simulink model "M_iHGU"  (R2019a)
settings: Solver=VariableStepAuto  StartTime=0.0  StopTime=10.0  RelTol=1e-3
undefined symbols (not defined in the file): ILC_B, M_iinfHGU_aD, M_iinfHGU_bD, M_iinfHGU_cD, M_iinfHGU_dD
settings Model: Creator=rache  LastModifiedBy=rache
settings DataIOCC: ReturnWorkspaceOutputs=off
settings DebuggingCC: ArithmeticOperatorsInVariantConditions=warning

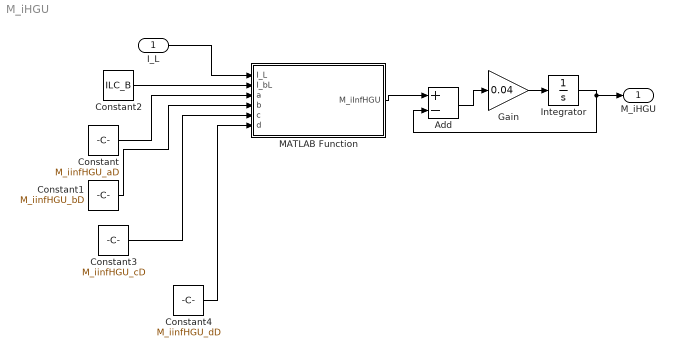
== system M_iHGU ==
  I_L : Inport
  Add : Sum  Inputs=+-
  Constant : Constant  Value=M_iinfHGU_aD
  Constant1 : Constant  Value=M_iinfHGU_bD
  Constant2 : Constant  Value=ILC_B
  Constant3 : Constant  Value=M_iinfHGU_cD
  Constant4 : Constant  Value=M_iinfHGU_dD
  Gain : Gain  Gain=0.04
  Integrator : Integrator
  MATLAB Function : MATLAB Function  TreatAsAtomicUnit=on
  M_iHGU : Outport
  wires:
  Integrator/1 -> Add/2, M_iHGU/1
  MATLAB Function/1(M_iInfHGU) -> Add/1
  Add/1 -> Gain/1
  Gain/1 -> Integrator/1
  Constant2/1 -> MATLAB Function/2(I_bL)
  I_L/1 -> MATLAB Function/1(I_L)
  Constant/1 -> MATLAB Function/3(a)
  Constant1/1 -> MATLAB Function/4(b)
  Constant3/1 -> MATLAB Function/5(c)
  Constant4/1 -> MATLAB Function/6(d)

== matlab function M_iHGU/MATLAB Function ==
  data: I_L input; M_iInfHGU output; I_bL input; a input; b input; c input; d input
function M_iInfHGU = fcn(I_L, I_bL, a, b, c, d)
M_iInfHGU = a+ b*tanh(c*I_L/I_bL + d);
